simulink model "MDM_v1"  (R2018b)
settings: Solver=VariableStepAuto  StartTime=0.0  StopTime=10.0  RelTol=1e-3
undefined symbols (not defined in the file): C1, C2, C3, C4, Cs, I2, I3, I4, I5, I6, I7, I8, Ie, Jr, k1, k2, k3, k4, k5, k6, k7, k8, R10, R3, R4, R5, R6, R7, R8, R9, Rb, Re
settings Model: Creator=HYJ  LastModifiedBy=HYJ

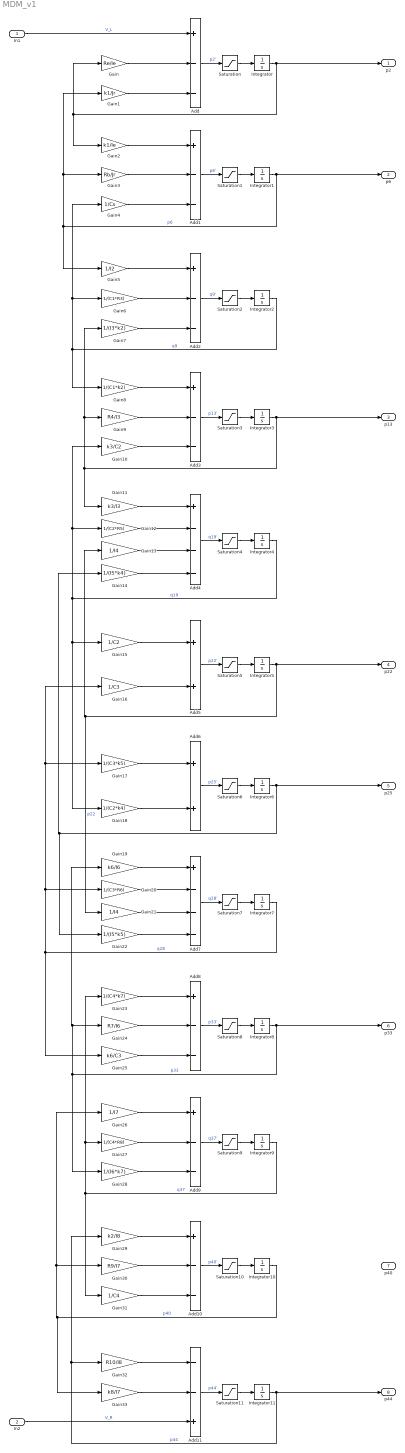
== system MDM_v1 ==
  In1 : Inport
  In2 : Inport  Port=2
  Add{,1..3,8..10} (7 alike) : Sum  Inputs=+--
  Add11 : Sum  Inputs=--+
  Add4 : Sum  Inputs=+---
  Add5 : Sum
  Add6 : Sum
  Add7 : Sum  Inputs=+---
  Gain : Gain  Gain=Re/Ie
  Gain1 : Gain  Gain=k1/Jr
  Gain10 : Gain  Gain=k3/C2
  Gain11 : Gain  Gain=k3/I3
  Gain12 : Gain  Gain=1/(C2*R5)
  Gain13 : Gain  Gain=1/I4
  Gain14 : Gain  Gain=1/(I5*k4)
  Gain15 : Gain  Gain=1/C2
  Gain16 : Gain  Gain=1/C3
  Gain17 : Gain  Gain=1/(C3*k5)
  Gain18 : Gain  Gain=1/(C2*k4)
  Gain19 : Gain  Gain=k6/I6
  Gain2 : Gain  Gain=k1/Ie
  Gain20 : Gain  Gain=1/(C3*R6)
  Gain21 : Gain  Gain=1/I4
  Gain22 : Gain  Gain=1/(I5*k5)
  Gain23 : Gain  Gain=1/(C4*k7)
  Gain24 : Gain  Gain=R7/I6
  Gain25 : Gain  Gain=k6/C3
  Gain26 : Gain  Gain=1/I7
  Gain27 : Gain  Gain=1/(C4*R8)
  Gain28 : Gain  Gain=1/(I6*k7)
  Gain29 : Gain  Gain=k2/I8
  Gain3 : Gain  Gain=Rb/Jr
  Gain30 : Gain  Gain=R9/I7
  Gain31 : Gain  Gain=1/C4
  Gain32 : Gain  Gain=R10/I8
  Gain33 : Gain  Gain=k8/I7
  Gain4 : Gain  Gain=1/Cs
  Gain5 : Gain  Gain=1/I2
  Gain6 : Gain  Gain=1/(C1*R3)
  Gain7 : Gain  Gain=1/(I3*k2)
  Gain8 : Gain  Gain=1/(C1*k2)
  Gain9 : Gain  Gain=R4/I3
  Integrator{,1..11} (12 alike) : Integrator
  Saturation{,1..11} (12 alike) : Saturate  UpperLimit=100  LowerLimit=-100
  p2 : Outport
  p6 : Outport  Port=2
  p13 : Outport  Port=3
  p22 : Outport  Port=4
  p25 : Outport  Port=5
  p33 : Outport  Port=6
  p40 : Outport  Port=7
  p44 : Outport  Port=8
  wires:
  Saturation/1 -> Integrator/1
  Add/1 -> Saturation/1  "p2'"
  In1/1 -> Add/1  "V_L"
  Gain/1 -> Add/2
  Gain1/1 -> Add/3
  Add1/1 -> Saturation1/1  "p6'"
  Saturation1/1 -> Integrator1/1
  Integrator1/1 -> p6/1, Gain5/1, Gain3/1, Gain1/1  "p6"
  Gain2/1 -> Add1/1
  Gain3/1 -> Add1/2
  Gain4/1 -> Add1/3
  Saturation2/1 -> Integrator2/1
  Add2/1 -> Saturation2/1  "q9'"
  Integrator2/1 -> Gain4/1, Gain6/1, Gain8/1  "q9"
  Gain6/1 -> Add2/2
  Gain7/1 -> Add2/3
  Gain5/1 -> Add2/1
  Gain8/1 -> Add3/1
  Add3/1 -> Saturation3/1  "p13'"
  Gain9/1 -> Add3/2
  Saturation3/1 -> Integrator3/1
  Gain10/1 -> Add3/3
  Add4/1 -> Saturation4/1  "q19'"
  Gain13/1 -> Add4/3
  Saturation4/1 -> Integrator4/1
  Gain12/1 -> Add4/2
  Integrator4/1 -> Gain18/1, Gain15/1, Gain12/1, Gain10/1  "q19"
  Gain11/1 -> Add4/1
  Gain14/1 -> Add4/4
  Saturation5/1 -> Integrator5/1
  Add5/1 -> Saturation5/1  "p22'"
  Integrator5/1 -> p22/1, Gain21/1, Gain13/1  "p22"
  Gain15/1 -> Add5/1
  Gain16/1 -> Add5/2
  Add6/1 -> Saturation6/1  "p25'"
  Saturation6/1 -> Integrator6/1
  Gain17/1 -> Add6/1
  Gain18/1 -> Add6/2
  Gain22/1 -> Add7/4
  Gain21/1 -> Add7/3
  Gain19/1 -> Add7/1
  Saturation7/1 -> Integrator7/1
  Add7/1 -> Saturation7/1  "q28'"
  Gain20/1 -> Add7/2
  Integrator7/1 -> Gain25/1, Gain20/1, Gain16/1, Gain17/1  "q28"
  Add8/1 -> Saturation8/1  "p33'"
  Gain25/1 -> Add8/3
  Saturation8/1 -> Integrator8/1
  Gain24/1 -> Add8/2
  Gain23/1 -> Add8/1
  Integrator8/1 -> p33/1, Gain28/1, Gain24/1, Gain19/1  "p33"
  Add9/1 -> Saturation9/1  "q37'"
  Gain27/1 -> Add9/2
  Saturation9/1 -> Integrator9/1
  Gain28/1 -> Add9/3
  Gain26/1 -> Add9/1
  Integrator9/1 -> Gain31/1, Gain23/1, Gain27/1  "q37"
  Saturation10/1 -> Integrator10/1
  Add10/1 -> Saturation10/1  "p40'"
  Gain29/1 -> Add10/1
  Gain30/1 -> Add10/2
  Gain31/1 -> Add10/3
  Integrator10/1 -> Gain33/1, Gain26/1, Gain30/1  "p40"
  Add11/1 -> Saturation11/1  "p44'"
  Saturation11/1 -> Integrator11/1
  In2/1 -> Add11/3  "V_R"
  Gain32/1 -> Add11/1
  Gain33/1 -> Add11/2
  Integrator/1 -> p2/1, Gain2/1, Gain/1
  Integrator3/1 -> p13/1, Gain9/1, Gain7/1, Gain11/1
  Integrator6/1 -> p25/1, Gain22/1, Gain14/1
  ? -> p40/1  "p40"
  Integrator11/1 -> p44/1, Gain29/1, Gain32/1  "p44"
